simulink subsystem "IMU"  (R2025b)
settings: Solver=VariableStepAuto  StartTime=0.0  StopTime=10.0  RelTol=1e-3
settings Model: Creator=JesseJabezArendse  LastModifiedBy=JesseJabezArendse
settings RTWCC: GPUComputeCapability=3.5

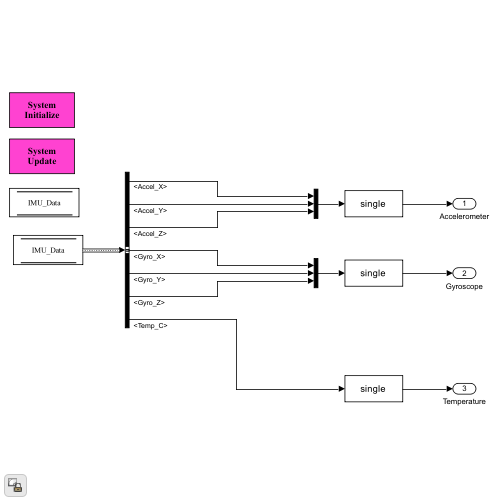
[thumbnail: Simulink's stored preview of the top-level diagram]
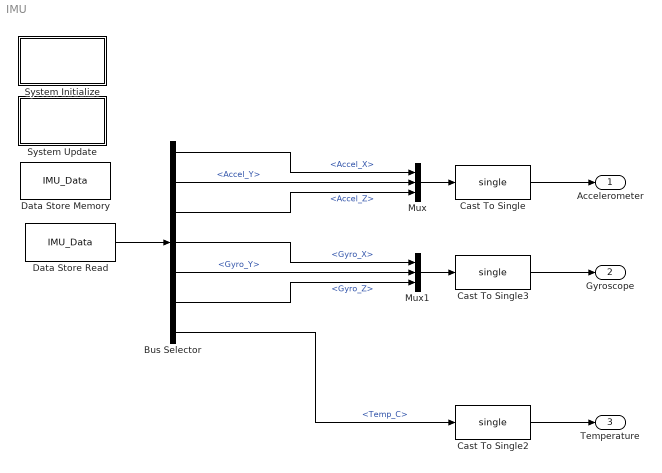
== system IMU ==
  Bus Selector : BusSelector  OutputSignals=Accel_X,Accel_Y,Accel_Z,Gyro_X,Gyro_Y,Gyro_Z,Temp_C
  Cast To Single : DataTypeConversion  OutDataTypeStr=single  SaturateOnIntegerOverflow=off  RndMeth=Floor
  Cast To Single2 : DataTypeConversion  OutDataTypeStr=single  SaturateOnIntegerOverflow=off  RndMeth=Floor
  Cast To Single3 : DataTypeConversion  OutDataTypeStr=single  SaturateOnIntegerOverflow=off  RndMeth=Floor
  Data Store Memory : DataStoreMemory  DataStoreName=IMU_Data  WriteAfterWriteMsg=warning  ShowAdditionalParam=off  OutDataTypeStr=Bus: IMU_t
  Data Store Read : DataStoreRead  DataStoreName=IMU_Data  IndexOptions=Index vector (dialog)  Indices=1  OutputSizes=1
  Mux : Mux  Inputs=3
  Mux1 : Mux  Inputs=3
  System Initialize : Subsystem  mask(System Initialize){ShowInLibBrowser=0}
      mask prompts: ShowInLibBrowser "Simulink:masks:CustCodeMaskParam1_MP"
      settings: CopyFcn=cccopyfcn(gcb)  OpenFcn=ccopenfcn('System Initialize Function')
      mask Help: eval('feval(''rtwprivate'',''rtwhelpview'',''rtw_sys_initialize_block'')');
      mask Display: disp('System\nInitialize');
  System Update : Subsystem  mask(System Update){ShowInLibBrowser=0}
      mask prompts: ShowInLibBrowser "Simulink:masks:CustCodeMaskParam1_MP"
      settings: CopyFcn=cccopyfcn(gcb)  OpenFcn=ccopenfcn('System Update Function')
      mask Help: eval('feval(''rtwprivate'',''rtwhelpview'',''rtw_sys_update_block'')');
      mask Display: disp('System\nUpdate');
  Accelerometer : Outport  OutDataTypeStr=single  PortDimensions=3
  Gyroscope : Outport  Port=2  OutDataTypeStr=single  PortDimensions=3
  Temperature : Outport  Port=3  OutDataTypeStr=single  PortDimensions=1
  wires:
  Cast To Single/1 -> Accelerometer/1
  Cast To Single2/1 -> Temperature/1
  Mux/1 -> Cast To Single/1
  Data Store Read/1 -> Bus Selector/1
  Bus Selector/7 -> Cast To Single2/1  "<Temp_C>"
  Bus Selector/1 -> Mux/1  "<Accel_X>"
  Bus Selector/2 -> Mux/2  "<Accel_Y>"
  Bus Selector/3 -> Mux/3  "<Accel_Z>"
  Bus Selector/6 -> Mux1/3  "<Gyro_Z>"
  Bus Selector/5 -> Mux1/2  "<Gyro_Y>"
  Mux1/1 -> Cast To Single3/1
  Bus Selector/4 -> Mux1/1  "<Gyro_X>"
  Cast To Single3/1 -> Gyroscope/1

== system IMU/System Initialize ==

== system IMU/System Update ==
